simulink model "ff"  (R2023a)
settings: Solver=VariableStepAuto  StartTime=0.0  StopTime=10.0  RelTol=1e-3
libraries: simulink_extras x5
settings Model: Creator=prath  LastModifiedBy=prath

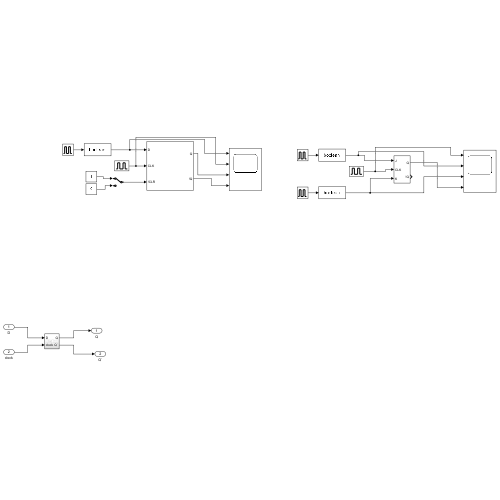
[thumbnail: Simulink's stored preview of the top-level diagram]
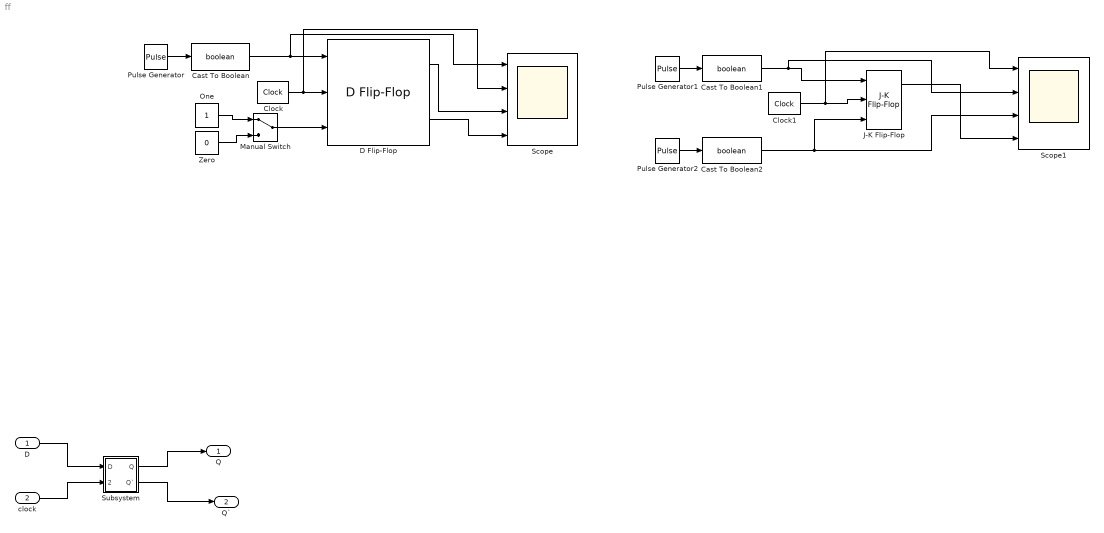
== system ff ==
  D : Inport
  clock : Inport  Port=2
  Cast To Boolean : DataTypeConversion  OutDataTypeStr=boolean  SaturateOnIntegerOverflow=off  RndMeth=Floor
  Cast To Boolean1 : DataTypeConversion  OutDataTypeStr=boolean  SaturateOnIntegerOverflow=off  RndMeth=Floor
  Cast To Boolean2 : DataTypeConversion  OutDataTypeStr=boolean  SaturateOnIntegerOverflow=off  RndMeth=Floor
  Clock : simulink_extras/Flip Flops/Clock  period=1
  Clock1 : simulink_extras/Flip Flops/Clock  period=1
  D Flip-Flop : simulink_extras/Flip Flops/D Flip-Flop
  J-K Flip-Flop : simulink_extras/Flip Flops/J-K Flip-Flop  initial_condition=0
  Manual Switch : ManualSwitch
  One : Constant  OutDataTypeStr=boolean
  Pulse Generator : DiscretePulseGenerator  PulseType=Time based  PulseWidth=50
  Pulse Generator1 : DiscretePulseGenerator  PulseType=Time based  PulseWidth=50
  Pulse Generator2 : DiscretePulseGenerator  PulseType=Time based  Period=4  PulseWidth=50
  Scope : Scope  NumInputPorts=4
  Scope1 : Scope  NumInputPorts=4
  Subsystem : Subsystem
  Zero : Constant  Value=0  OutDataTypeStr=boolean
  Q : Outport
  Q` : Outport  Port=2
  wires:
  Manual Switch/1 -> D Flip-Flop/3
  One/1 -> Manual Switch/1
  Zero/1 -> Manual Switch/2
  D Flip-Flop/1 -> Scope/3
  D Flip-Flop/2 -> Scope/4
  Clock/1 -> Scope/2, D Flip-Flop/2
  Cast To Boolean/1 -> Scope/1, D Flip-Flop/1
  Pulse Generator/1 -> Cast To Boolean/1
  Clock1/1 -> Scope1/1, J-K Flip-Flop/2
  Pulse Generator1/1 -> Cast To Boolean1/1
  Cast To Boolean1/1 -> Scope1/2, J-K Flip-Flop/1
  Pulse Generator2/1 -> Cast To Boolean2/1
  Cast To Boolean2/1 -> Scope1/3, J-K Flip-Flop/3
  J-K Flip-Flop/1 -> Scope1/4
  D/1 -> Subsystem/1(D)
  clock/1 -> Subsystem/2(clock)
  Subsystem/1(Q) -> Q/1
  Subsystem/2(Q`) -> Q`/1

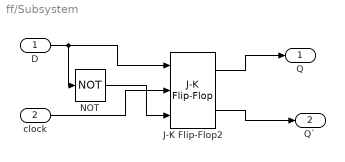
== system ff/Subsystem ==
  D : Inport
  clock : Inport  Port=2
  J-K Flip-Flop2 : simulink_extras/Flip Flops/J-K Flip-Flop  initial_condition=0
  NOT : Logic  Operator=NOT  IconShape=distinctive  AllPortsSameDT=off  OutDataTypeStr=boolean
  Q : Outport
  Q` : Outport  Port=2
  wires:
  J-K Flip-Flop2/1 -> Q/1
  NOT/1 -> J-K Flip-Flop2/3
  D/1 -> NOT/1, J-K Flip-Flop2/1
  clock/1 -> J-K Flip-Flop2/2
  J-K Flip-Flop2/2 -> Q`/1
